simulink model "lab10"  (R2022b)
settings: Solver=VariableStepAuto  StartTime=0.0  StopTime=10.0  RelTol=1e-3
settings Model: Creator=jakes  LastModifiedBy=jakes

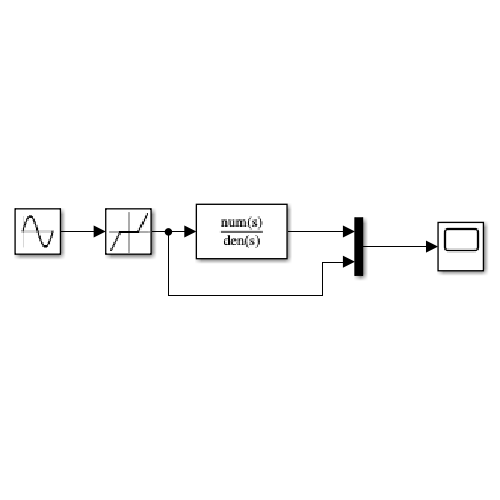
[thumbnail: Simulink's stored preview of the top-level diagram]
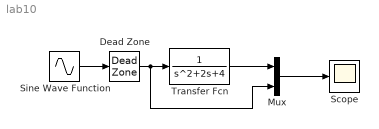
== system lab10 ==
  Dead Zone : DeadZone
  Mux : Mux  Inputs=2
  Scope : Scope
  Sine Wave Function : Sin  Frequency=1.4  SampleTime=0
  Transfer Fcn : TransferFcn  Denominator=[1,2,4]
  wires:
  Sine Wave Function/1 -> Dead Zone/1
  Transfer Fcn/1 -> Mux/1
  Dead Zone/1 -> Mux/2, Transfer Fcn/1
  Mux/1 -> Scope/1
